simulink model "scheme16_8"  (R2019a)
settings: Solver=VariableStepAuto  StartTime=0.0  StopTime=200  FixedStep=1e-3  MaxStep=1e-3  RelTol=1e-3  EnableMultiTasking=on
values from neighbouring files (symbols this model uses):
  G = ss(G)    [main16_8.m]
  mu = 16    [main16_8.m]
  X0 = 1    [main16_8.m]
settings Model: Creator=Adriano  LastModifiedBy=adria
settings DataIOCC: LimitDataPoints=on  SaveFormat=Array  ReturnWorkspaceOutputs=off
settings OptimizationCC: LifeSpan=inf
settings DebuggingCC: SFUnexpectedBacktrackingDiag=warning  SFNoUnconditionalDefaultTransitionDiag=warning  SFExecutionAtInitializationDiag=none  ArithmeticOperatorsInVariantConditions=warning
settings HardwareCC: ProdBitPerPointer=32  ProdBitPerSizeT=32  ProdBitPerPtrDiffT=32  ProdLargestAtomicFloat=None  ProdIntDivRoundTo=Undefined  ProdEndianess=Unspecified  ProdWordSize=32  ProdHWDeviceType=32-bit Generic
settings ModelReferenceCC: PropagateSignalLabelsOutOfModel=off
settings SFSimCC: SimUseLocalCustomCode=off
settings RTWCC: RTWUseLocalCustomCode=off
settings CodeAppCC: StateflowObjectComments=on
settings GRTTargetCC: TargetLangStandard=C89/C90 (ANSI)  GeneratePreprocessorConditionals=Disable all
settings ConfigComp: CovMetricSettings=dw  CovHtmlReporting=on  CovSaveCumulativeToWorkspaceVar=on  CovSaveSingleToWorkspaceVar=on  CovExternalEMLEnable=off

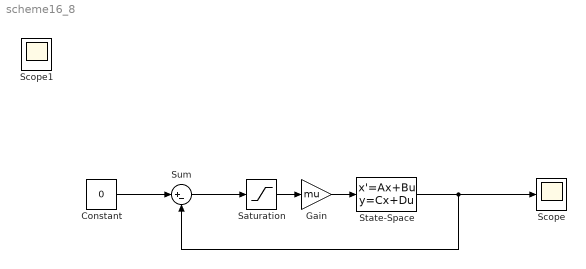
== system scheme16_8 ==
  Constant : Constant  Value=0
  Gain : Gain  Gain=mu
  Saturation : Saturate  UpperLimit=X0  LowerLimit=-X0
  Scope : Scope
  State-Space : StateSpace  A=G.a  B=G.b  C=G.c  D=G.d  InitialCondition=[1 1 1]
  Sum : Sum  Inputs=|+-
  Scope1 : Scope
  wires:
  Constant/1 -> Sum/1
  Sum/1 -> Saturation/1
  Saturation/1 -> Gain/1
  State-Space/1 -> Scope/1, Sum/2
  Gain/1 -> State-Space/1
